simulink model "myPendulum"  (R2022b)
settings: Solver=VariableStepAuto  StartTime=0.0  StopTime=20  RelTol=1e-3
values from neighbouring files (symbols this model uses):
  d0 = 1    [mainForProject.m]
  d1 = 1    [mainForProject.m]
  delayVal = 0.02    [mainForProject.m]
  denCtrlFinal = denCtrl1    [mainForProject.m]
  denCtrlRef = cell2mat(denCtrlRef)    [mainForProject.m]
  denFfctrl = cell2mat(denFfctrl)    [mainForProject.m]
  finalAngle = 2 * pi    (= 6.28318530718)    [mainForProject.m]
  forceSaturation = 100    [mainForProject.m]
  initAngle = pi    (= 3.14159265359)    [mainForProject.m]
  noiseFrequency = 100    [mainForProject.m]
  noisePower = 10    [mainForProject.m]
  numCtrlFinal = numCtrl1    [mainForProject.m]
  numCtrlRef = cell2mat(numCtrlRef)    [mainForProject.m]
  numFfctrl = cell2mat(numFfctrl)    [mainForProject.m]
libraries: simulink x1
settings Model: Creator=utente  LastModifiedBy=utente
settings SolverCC: ZeroCrossAlgorithm=Adaptive
settings DebuggingCC: IgnoredZcDiagnostic=none

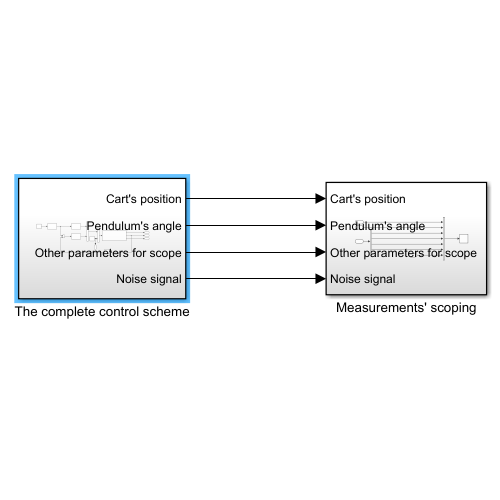
[thumbnail: Simulink's stored preview of the top-level diagram]
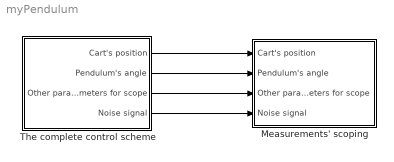
== system myPendulum ==
  Measurements' scoping : Subsystem
  The complete control scheme : Subsystem
  wires:
  The complete control scheme/3(Other parameters for scope) -> Measurements' scoping/3(Other parameters for scope)
  The complete control scheme/2(Pendulum's angle) -> Measurements' scoping/2(Pendulum's angle)
  The complete control scheme/1(Cart's position) -> Measurements' scoping/1(Cart's position)
  The complete control scheme/4(Noise signal) -> Measurements' scoping/4(Noise signal)

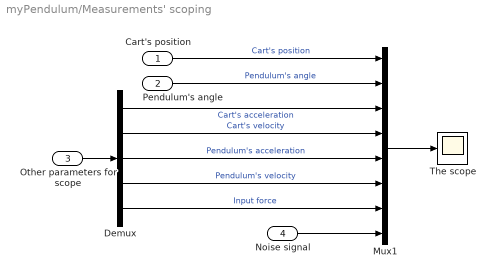
== system myPendulum/Measurements' scoping ==
  Cart's position : Inport
  Pendulum's angle : Inport  Port=2
  Other parameters for scope : Inport  Port=3
  Noise signal : Inport  Port=4
  Demux : Demux  Outputs=5
  Mux1 : Mux  Inputs=8
  The scope : Scope
  wires:
  Mux1/1 -> The scope/1
  Demux/3 -> Mux1/5  "Pendulum's acceleration"
  Demux/2 -> Mux1/4  "Cart's velocity"
  Demux/4 -> Mux1/6  "Pendulum's velocity"
  Demux/1 -> Mux1/3  "Cart's acceleration"
  Other parameters for scope/1 -> Demux/1
  Cart's position/1 -> Mux1/1  "Cart's position"
  Pendulum's angle/1 -> Mux1/2  "Pendulum's angle"
  Noise signal/1 -> Mux1/8
  Demux/5 -> Mux1/7  "Input force"

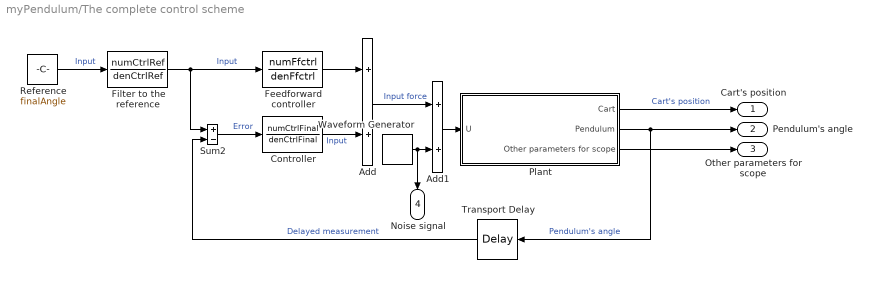
== system myPendulum/The complete control scheme ==
  Add : Sum
  Add1 : Sum
  Controller : TransferFcn  Numerator=numCtrlFinal  Denominator=denCtrlFinal
  Feedforward controller : TransferFcn  Numerator=numFfctrl  Denominator=denFfctrl
  Filter to the reference : TransferFcn  Numerator=numCtrlRef  Denominator=denCtrlRef
  Plant : Subsystem  mask(Inverted pendulum on cart){Mcart=0.455, m=0.21, l=0.61/2, g=9.8}
      mask prompts: Mcart "Mass of cart (kg):"; m "Mass of pendulum (kg):"; l "Distance to pendulum center of mass(m):"; g "Acceleration of gravity (m/s^2):"
      mask help: Unmask and double-click to see dynamics
      mask Help: Nonlinear dynamics of inverted pendulum on cart.
  Reference : Constant  Value=finalAngle
  Sum2 : Sum  Inputs=+-  InputSameDT=on  SaturateOnIntegerOverflow=on  OutDataTypeStr=Inherit: Same as first input
  Transport Delay : TransportDelay  DelayTime=delayVal
  Waveform Generator : simulink/Sources/Waveform Generator  OutMin=[]  OutMax=[]  OutDataTypeStr=double  SelectedSignal=1  Signals=sin(noisePower, noiseFrequency, 0)  BlockNames=MultiportSwitch_f456f3024f9a455  SampleTime=0.1
  Cart's position : Outport
  Pendulum's angle : Outport  Port=2
  Other parameters for scope : Outport  Port=3
  Noise signal : Outport  Port=4
  wires:
  Reference/1 -> Filter to the reference/1  "Input"
  Plant/1(Cart) -> Cart's position/1  "Cart's position"
  Transport Delay/1 -> Sum2/2  "Delayed measurement"
  Add/1 -> Add1/1  "Input force"
  Plant/3(Other parameters for scope) -> Other parameters for scope/1
  Plant/2(Pendulum) -> Transport Delay/1, Pendulum's angle/1  "Pendulum's angle"
  Sum2/1 -> Controller/1  "Error"
  Feedforward controller/1 -> Add/1
  Controller/1 -> Add/2  "Input"
  Filter to the reference/1 -> Feedforward controller/1, Sum2/1  "Input"
  Waveform Generator/1 -> Noise signal/1, Add1/2
  Add1/1 -> Plant/1(U)

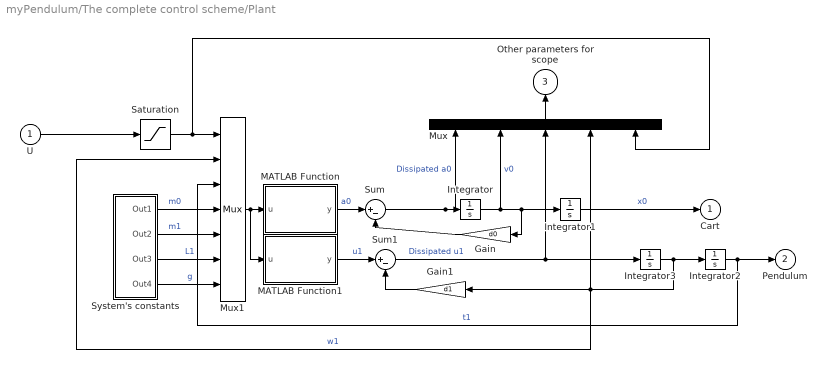
== system myPendulum/The complete control scheme/Plant ==
  U : Inport
  Gain : Gain  Gain=d0
  Gain1 : Gain  Gain=d1
  Integrator : Integrator
  Integrator1 : Integrator
  Integrator2 : Integrator  InitialCondition=initAngle
  Integrator3 : Integrator
  MATLAB Function : MATLAB Function  TreatAsAtomicUnit=on
  MATLAB Function1 : MATLAB Function  TreatAsAtomicUnit=on
  Mux : Mux  Inputs=5
  Mux1 : Mux  Inputs=7
  Saturation : Saturate  UpperLimit=forceSaturation  LowerLimit=-forceSaturation
  Sum : Sum  Inputs=|+-
  Sum1 : Sum  Inputs=|+-
  System's constants : Subsystem
  Cart : Outport  InitialOutput=0  VectorParamsAs1DForOutWhenUnconnected=off
  Pendulum : Outport  Port=2  InitialOutput=0  VectorParamsAs1DForOutWhenUnconnected=off
  Other parameters for scope : Outport  Port=3
  wires:
  Integrator3/1 -> Gain1/1, Mux/4, Mux1/2, Integrator2/1  "w1"
  Integrator2/1 -> Mux1/3, Pendulum/1  "t1"
  System's constants/1(Out1) -> Mux1/4  "m0"
  System's constants/2(Out2) -> Mux1/5  "m1"
  System's constants/3(Out3) -> Mux1/6  "L1"
  System's constants/4(Out4) -> Mux1/7  "g"
  Mux1/1 -> MATLAB Function/1(u), MATLAB Function1/1(u)
  Integrator1/1 -> Cart/1  "x0"
  Integrator/1 -> Gain/1, Integrator1/1, Mux/2  "v0"
  U/1 -> Saturation/1
  Mux/1 -> Other parameters for scope/1
  Saturation/1 -> Mux/5, Mux1/1
  MATLAB Function/1(y) -> Sum/1  "a0"
  Sum/1 -> Integrator/1, Mux/1  "Dissipated a0"
  Gain/1 -> Sum/2
  Sum1/1 -> Integrator3/1, Mux/3  "Dissipated u1"
  MATLAB Function1/1(y) -> Sum1/1  "u1"
  Gain1/1 -> Sum1/2

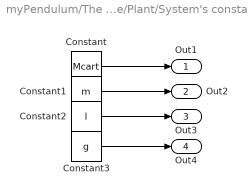
== system myPendulum/The complete control scheme/Plant/System's constants ==
  Constant : Constant  Value=Mcart
  Constant1 : Constant  Value=m
  Constant2 : Constant  Value=l
  Constant3 : Constant  Value=g
  Out1 : Outport
  Out2 : Outport  Port=2
  Out3 : Outport  Port=3
  Out4 : Outport  Port=4
  wires:
  Constant/1 -> Out1/1
  Constant1/1 -> Out2/1
  Constant2/1 -> Out3/1
  Constant3/1 -> Out4/1

== matlab function myPendulum/The complete control scheme/Plant/MATLAB Function ==
  data: u input; y output
function y = a0Calculate(u)
    %% Parametri desiderati : 
    % J1,L1,G,INFORCE,M0,M1,PENDVEL,PENDPOS
    y = double(a0Funct(1 / 3 * u(5) * u(6) ^ 2,u(6), u(7), u(1), u(4), u(5), u(2), u(3)));
end

== matlab function myPendulum/The complete control scheme/Plant/MATLAB Function1 ==
  data: u input; y output
function y = u1Calculate(u)
    %% Parametri desiderati : 
    % J1,L1,G,INFORCE,M0,M1,PENDVEL,PENDPOS
    y = double(u1Funct(1 / 3 * u(5) * u(6) ^ 2,u(6), u(7), u(1), u(4), u(5), u(2), u(3)));
end
